simulink model "FYP_Flywheel_Stage3_DCServo"  (R2024a)
settings: Solver=ode45  StartTime=0.0  StopTime=10  RelTol=1e-3
values from neighbouring files (symbols this model uses):
  B = 1.0e-3    (= 0.001)    [FYP_Flywheel_Stage2_build.m]    (also in FYP_Flywheel_Stage3_DCServo_build.m; FYP_Flywheel_Stage4_v2_StableClosedLoop_build.m; FYP_Flywheel_Stage5_COMPLETE_v2.m)
  J_total = Jm + Jf    (= 0.51)    [FYP_Flywheel_Stage3_DCServo_build.m]    (also in FYP_Flywheel_Stage4_v2_StableClosedLoop_build.m; FYP_Flywheel_Stage5_COMPLETE_v2.m)
  Jf = 0.50    (= 0.5)    [FYP_Flywheel_Stage3_DCServo_build.m]    (also in FYP_Flywheel_Stage4_v2_StableClosedLoop_build.m; FYP_Flywheel_Stage5_COMPLETE_v2.m)
  Ke = 0.05    [FYP_Flywheel_Stage3_DCServo_build.m]    (also in FYP_Flywheel_Stage4_v2_StableClosedLoop_build.m; FYP_Flywheel_Stage5_COMPLETE_v2.m)
  Kt = 0.05    [FYP_Flywheel_Stage3_DCServo_build.m]    (also in FYP_Flywheel_Stage4_v2_StableClosedLoop_build.m; FYP_Flywheel_Stage5_COMPLETE_v2.m)
  L = 0.02    [FYP_Flywheel_Stage3_DCServo_build.m]    (also in FYP_Flywheel_Stage4_v2_StableClosedLoop_build.m; FYP_Flywheel_Stage5_COMPLETE_v2.m)
  omega0 = 2*pi*n0/60    (= 314.159265359)    [FYP_Flywheel_Stage1_build.m]    (also in FYP_Flywheel_Stage2_build.m; FYP_Flywheel_Stage3_DCServo_build.m; FYP_Flywheel_Stage4_v2_StableClosedLoop_build.m; FYP_Flywheel_Stage5_COMPLETE_v2.m)
  R = 0.8    [FYP_Flywheel_Stage3_DCServo_build.m]    (also in FYP_Flywheel_Stage4_v2_StableClosedLoop_build.m; FYP_Flywheel_Stage5_COMPLETE_v2.m)
  Tc = 0.05    [FYP_Flywheel_Stage2_build.m]    (also in FYP_Flywheel_Stage3_DCServo_build.m; FYP_Flywheel_Stage4_v2_StableClosedLoop_build.m; FYP_Flywheel_Stage5_COMPLETE_v2.m)
settings Model: Creator=cheng  LastModifiedBy=cheng

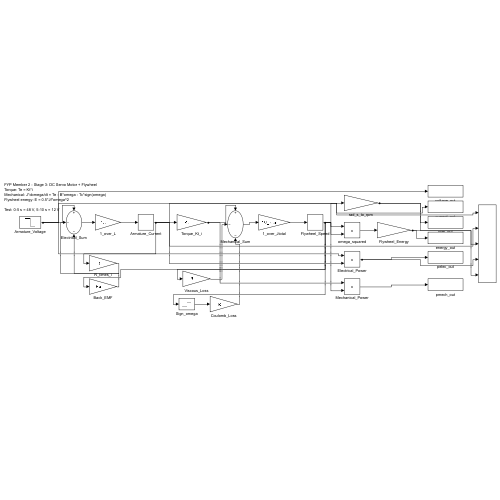
[thumbnail: Simulink's stored preview of the top-level diagram]
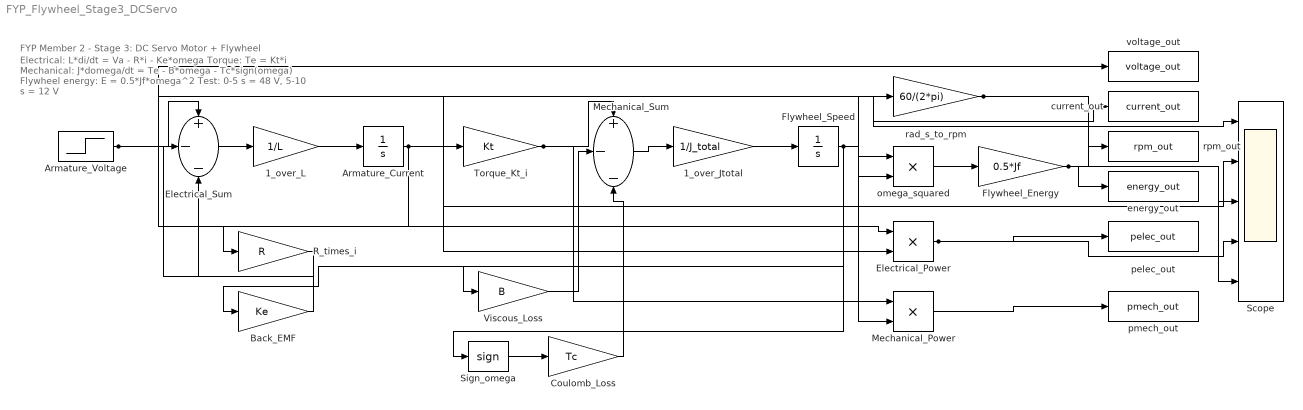
== system FYP_Flywheel_Stage3_DCServo ==
  note: FYP Member 2 - Stage 3: DC Servo Motor + Flywheel
  note: Electrical: L*di/dt = Va - R*i - Ke*omega
      | Torque: Te = Kt*i
      | Mechanical: J*domega/dt = Te - B*omega - Tc*sign(omega)
      | Flywheel energy: E = 0.5*Jf*omega^2
      |
      | Test: 0-5 s = 48 V, 5-10 s = 12 V
  1_over_Jtotal : Gain  Gain=1/J_total
  1_over_L : Gain  Gain=1/L
  Armature_Current : Integrator
  Armature_Voltage : Step  Time=5  Before=48  After=12  SampleTime=0
  Back_EMF : Gain  Gain=Ke
  Coulomb_Loss : Gain  Gain=Tc
  Electrical_Power : Product  Inputs=**
  Electrical_Sum : Sum  Inputs=+--
  Flywheel_Energy : Gain  Gain=0.5*Jf
  Flywheel_Speed : Integrator  InitialCondition=omega0
  Mechanical_Power : Product  Inputs=**
  Mechanical_Sum : Sum  Inputs=+--
  R_times_i : Gain  Gain=R
  Scope : Scope  NumInputPorts=5
  Sign_omega : Signum
  Torque_Kt_i : Gain  Gain=Kt
  Viscous_Loss : Gain  Gain=B
  current_out : ToWorkspace  VariableName=current_out  SaveFormat=Timeseries  SampleTime=-1
  energy_out : ToWorkspace  VariableName=energy_out  SaveFormat=Timeseries  SampleTime=-1
  omega_squared : Product  Inputs=**
  pelec_out : ToWorkspace  VariableName=pelec_out  SaveFormat=Timeseries  SampleTime=-1
  pmech_out : ToWorkspace  VariableName=pmech_out  SaveFormat=Timeseries  SampleTime=-1
  rad_s_to_rpm : Gain  Gain=60/(2*pi)
  rpm_out : ToWorkspace  VariableName=rpm_out  SaveFormat=Timeseries  SampleTime=-1
  voltage_out : ToWorkspace  VariableName=voltage_out  SaveFormat=Timeseries  SampleTime=-1
  wires:
  Armature_Voltage/1 -> Electrical_Sum/1, Electrical_Power/1, voltage_out/1, Scope/1
  Electrical_Sum/1 -> 1_over_L/1
  1_over_L/1 -> Armature_Current/1
  Armature_Current/1 -> R_times_i/1, Torque_Kt_i/1, Electrical_Power/2, current_out/1, Scope/2
  R_times_i/1 -> Electrical_Sum/2
  Torque_Kt_i/1 -> Mechanical_Sum/1, Mechanical_Power/1
  Mechanical_Sum/1 -> 1_over_Jtotal/1
  1_over_Jtotal/1 -> Flywheel_Speed/1
  Flywheel_Speed/1 -> Back_EMF/1, Viscous_Loss/1, Sign_omega/1, rad_s_to_rpm/1, omega_squared/1, omega_squared/2, Mechanical_Power/2
  Back_EMF/1 -> Electrical_Sum/3
  Viscous_Loss/1 -> Mechanical_Sum/2
  Sign_omega/1 -> Coulomb_Loss/1
  Coulomb_Loss/1 -> Mechanical_Sum/3
  omega_squared/1 -> Flywheel_Energy/1
  rad_s_to_rpm/1 -> rpm_out/1, Scope/3
  Flywheel_Energy/1 -> energy_out/1, Scope/5
  Electrical_Power/1 -> pelec_out/1, Scope/4
  Mechanical_Power/1 -> pmech_out/1
